simulink model "model2_2016a"  (R2016a)
settings: Solver=ode4  StartTime=0.0  StopTime=60  FixedStep=0.01  RelTol=1e-3
values from neighbouring files (symbols this model uses):
  D1 = par(2)    [cel.m]    (also in cel_P.m; cel_PD2.m = 38.2416; dane.m; dane.mat = 35.0184631454)
  D2 = par(4)    [cel.m]    (also in cel_P.m; cel_PD2.m = par(2); cel_z.m = par(2); dane.m)
  I3 = par(6)    [cel.m]    (also in cel_PD2.m = 0.0358; cel_bezFeedforward.m = par(2); dane.m; dane.mat = 0.0341130667622)
  Ko = 2    [dane.m]    (also in dane.mat = 10; dane2.mat = 10; dane3.mat = 10; dane4.mat = 10)
  Kr = par(7)    [cel.m]    (also in cel_P.m = par(5); cel_PD2.m = 0.3949; cel_bezFeedforward.m = par(3); dane.m = 3)
  Kw1 = 2    [dane.m]    (also in dane.mat = 10; dane2.mat = 10; dane3.mat = 10; dane4.mat = 10)
  Kw2 = 3    [dane.m]    (also in dane.mat = 5; dane2.mat = 5; dane3.mat = 5; dane4.mat = 5)
  limit2 = 10    [dane.m]    (also in dane.mat = 40; dane2.mat = 40; dane3.mat = 40; dane4.mat = 40)
  P1 = par(1)    [cel.m]    (also in cel_P.m; cel_PD2.m = 0.0302; dane.m; dane.mat = 0.804768322622)
  P2 = par(3)    [cel.m]    (also in cel_P.m; cel_PD2.m = par(1); cel_z.m = par(1); dane.m)
  P3 = par(5)    [cel.m]    (also in cel_PD2.m = 6.71669750093e-06; cel_bezFeedforward.m = par(1); dane.m; dane.mat = 3.3559799843e-06)
  r = 3    [dane.m]    (also in dane.mat = 50; dane2.mat = 20; dane3.mat = 70; dane4.mat = 70)
  tau = 0    [dane.m]    (also in dane.mat = 1; dane2.mat = 1; dane3.mat = 1; dane4.mat = 1)
  To = 2    [dane.m]    (also in dane.mat = 1; dane2.mat = 1; dane3.mat = 1; dane4.mat = 1)
  Tw2 = .1    (= 0.1)    [dane.m]    (also in dane.mat; dane2.mat; dane3.mat; dane4.mat)
undefined symbols (not defined in the file or in its folder): sigbuilder_block
libraries: simulink x2
settings Model: Creator=Maciek  LastModifiedBy=Daniel Rubak
settings GRTTargetCC: GeneratePreprocessorConditionals=Use local settings

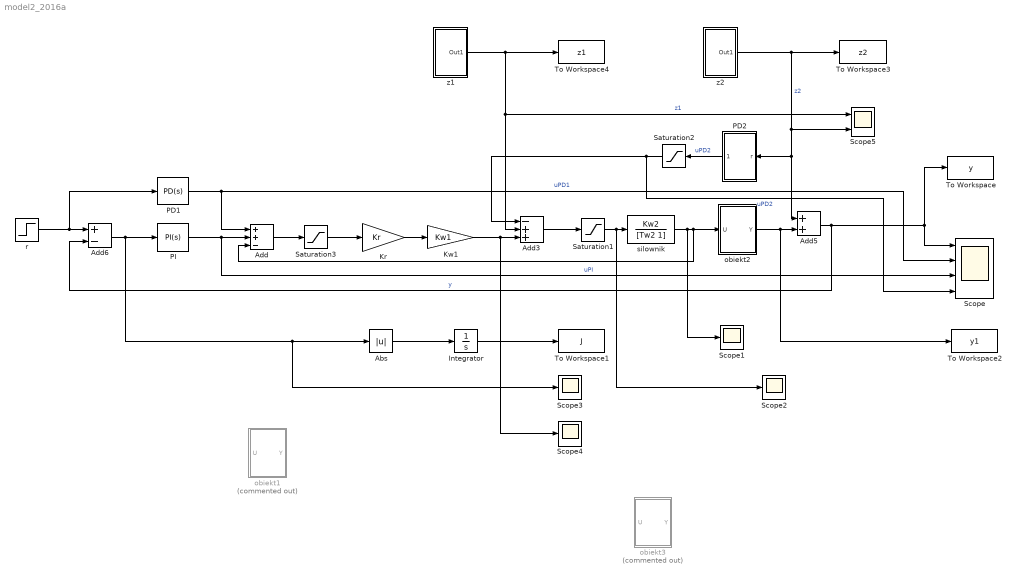
== system model2_2016a ==
  Abs : Abs
  Add : Sum  Inputs=++-
  Add3 : Sum  Inputs=-++
  Add5 : Sum
  Add6 : Sum  Inputs=+-
  Integrator : Integrator
  Kr : Gain  Gain=Kr
  "Kw1 " : Gain  Gain=Kw1
  PD1 : simulink/Continuous/PID Controller  Controller=PD  TimeDomain=Continuous-time  SampleTime=-1  IntegratorMethod=Forward Euler  FilterMethod=Forward Euler  Form=Parallel  UseFilter=on  ControllerParametersSource=internal  P=P1  I=1  D=D1  N=100  InitialConditionSource=internal  InitialConditionForIntegrator=0  InitialConditionForFilter=0  ExternalReset=none  LimitOutput=on  UpperSaturationLimit=limit2  LowerSaturationLimit=-limit2  LinearizeAsGain=on  AntiWindupMode=none  Kb=1  TrackingMode=off  Kt=1  PParamMin=[]  PParamMax=[]  IParamMin=[]  IParamMax=[]  DParamMin=[]  DParamMax=[]  NParamMin=[]  NParamMax=[]  KbParamMin=[]  KbParamMax=[]  KtParamMin=[]  KtParamMax=[]  POutMin=[]  POutMax=[]  IOutMin=[]  IOutMax=[]  DOutMin=[]  DOutMax=[]  NOutMin=[]  NOutMax=[]  KbOutMin=[]  KbOutMax=[]  KtOutMin=[]  KtOutMax=[]  IntegratorOutMin=[]  IntegratorOutMax=[]  FilterOutMin=[]  FilterOutMax=[]  SumOutMin=[]  SumOutMax=[]  SumI1OutMin=[]  SumI1OutMax=[]  SumI2OutMin=[]  SumI2OutMax=[]  SumI3OutMin=[]  SumI3OutMax=[]  SumDOutMin=[]  SumDOutMax=[]  SaturationOutMin=[]  SaturationOutMax=[]  IntegratorContinuousStateAttributes=''  IntegratorStateMustResolveToSignalObject=off  IntegratorRTWStateStorageClass=Auto  FilterContinuousStateAttributes=''  FilterStateMustResolveToSignalObject=off  FilterRTWStateStorageClass=Auto  DifferentiatorICPrevScaledInput=0  DifferentiatorOutMin=[]  DifferentiatorOutMax=[]
  PD2 : Subsystem
  PI : simulink/Continuous/PID Controller  Controller=PI  TimeDomain=Continuous-time  SampleTime=-1  IntegratorMethod=Forward Euler  FilterMethod=Forward Euler  Form=Parallel  UseFilter=on  ControllerParametersSource=internal  P=P3  I=I3  D=0  N=100  InitialConditionSource=internal  InitialConditionForIntegrator=0  InitialConditionForFilter=0  ExternalReset=none  LimitOutput=on  UpperSaturationLimit=limit2  LowerSaturationLimit=-limit2  LinearizeAsGain=on  AntiWindupMode=back-calculation  Kb=1/sqrt(max(0.001,I3))  TrackingMode=off  Kt=1  PParamMin=[]  PParamMax=[]  IParamMin=[]  IParamMax=[]  DParamMin=[]  DParamMax=[]  NParamMin=[]  NParamMax=[]  KbParamMin=[]  KbParamMax=[]  KtParamMin=[]  KtParamMax=[]  POutMin=[]  POutMax=[]  IOutMin=[]  IOutMax=[]  DOutMin=[]  DOutMax=[]  NOutMin=[]  NOutMax=[]  KbOutMin=[]  KbOutMax=[]  KtOutMin=[]  KtOutMax=[]  IntegratorOutMin=[]  IntegratorOutMax=[]  FilterOutMin=[]  FilterOutMax=[]  SumOutMin=[]  SumOutMax=[]  SumI1OutMin=[]  SumI1OutMax=[]  SumI2OutMin=[]  SumI2OutMax=[]  SumI3OutMin=[]  SumI3OutMax=[]  SumDOutMin=[]  SumDOutMax=[]  SaturationOutMin=[]  SaturationOutMax=[]  IntegratorContinuousStateAttributes=''  IntegratorStateMustResolveToSignalObject=off  IntegratorRTWStateStorageClass=Auto  FilterContinuousStateAttributes=''  FilterStateMustResolveToSignalObject=off  FilterRTWStateStorageClass=Auto  DifferentiatorICPrevScaledInput=0  DifferentiatorOutMin=[]  DifferentiatorOutMax=[]
  Saturation1 : Saturate  UpperLimit=limit2  LowerLimit=-limit2
  Saturation2 : Saturate  UpperLimit=20  LowerLimit=-20
  Saturation3 : Saturate  UpperLimit=limit2  LowerLimit=-limit2
  Scope : Scope  NumInputPorts=4
  Scope{1..4} (4 alike) : Scope
  Scope5 : Scope  NumInputPorts=2
  To Workspace : ToWorkspace  VariableName=y  SaveFormat=Timeseries  SampleTime=-1
  To Workspace1 : ToWorkspace  VariableName=J  SampleTime=-1
      settings: MaxDataPoints=1
  To Workspace2 : ToWorkspace  VariableName=y1  SaveFormat=Timeseries  SampleTime=-1
  To Workspace3 : ToWorkspace  VariableName=z2  SaveFormat=Timeseries  SampleTime=-1
  To Workspace4 : ToWorkspace  VariableName=z1  SaveFormat=Timeseries  SampleTime=-1
  obiekt1 : Subsystem  Commented=on
  obiekt2 : Subsystem
  obiekt3 : Subsystem  Commented=on
  r : Step  After=r  SampleTime=0
  silownik : TransferFcn  Numerator=Kw2  Denominator=[Tw2 1]
  z1 : Subsystem
  z2 : Subsystem
  wires:
  r/1 -> PD1/1, Add6/1
  PD1/1 -> Scope/2, Add/1  "uPD1"
  Kr/1 -> "Kw1 "/1
  PI/1 -> Add/2, Scope/3  "uPI"
  Add6/1 -> Scope3/1, Abs/1, PI/1
  Add5/1 -> Add6/2, To Workspace/1, Scope/1  "y"
  PD2/1(uPD2) -> Saturation2/1  "uPD2"
  obiekt2/1(Y) -> To Workspace2/1, Add5/2
  Integrator/1 -> To Workspace1/1
  Abs/1 -> Integrator/1
  Saturation1/1 -> Scope2/1, silownik/1
  Saturation2/1 -> Scope/4, Add3/1  "uPD2"
  Add3/1 -> Saturation1/1
  z1/1(Out1) -> Scope5/1, Add3/2, To Workspace4/1  "z1"
  z2/1(Out1) -> To Workspace3/1, Scope5/2, Add5/1, PD2/1(r)  "z2"
  "Kw1 "/1 -> Scope4/1, Add3/3
  Saturation3/1 -> Kr/1
  silownik/1 -> Scope1/1, obiekt2/1(U), Add/3
  Add/1 -> Saturation3/1

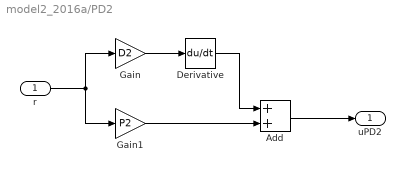
== system model2_2016a/PD2 ==
  r : Inport
  Add : Sum
  Derivative : Derivative
  Gain : Gain  Gain=D2
  Gain1 : Gain  Gain=P2
  uPD2 : Outport
  wires:
  Derivative/1 -> Add/1
  Gain1/1 -> Add/2
  r/1 -> Gain/1, Gain1/1
  Gain/1 -> Derivative/1
  Add/1 -> uPD2/1

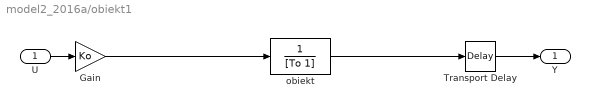
== system model2_2016a/obiekt1 ==
  U : Inport
  Gain : Gain  Gain=Ko
  Transport Delay : TransportDelay  DelayTime=tau
  obiekt : TransferFcn  Numerator=1  Denominator=[To 1]
  Y : Outport
  wires:
  U/1 -> Gain/1
  Gain/1 -> obiekt/1
  Transport Delay/1 -> Y/1
  obiekt/1 -> Transport Delay/1

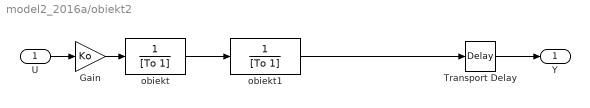
== system model2_2016a/obiekt2 ==
  U : Inport
  Gain : Gain  Gain=Ko
  Transport Delay : TransportDelay  DelayTime=tau
  obiekt : TransferFcn  Numerator=1  Denominator=[To 1]
  obiekt1 : TransferFcn  Numerator=1  Denominator=[To 1]
  Y : Outport
  wires:
  U/1 -> Gain/1
  Gain/1 -> obiekt/1
  obiekt/1 -> obiekt1/1
  Transport Delay/1 -> Y/1
  obiekt1/1 -> Transport Delay/1

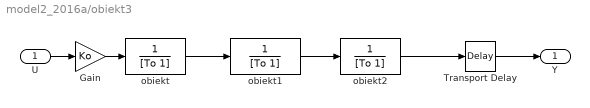
== system model2_2016a/obiekt3 ==
  U : Inport
  Gain : Gain  Gain=Ko
  Transport Delay : TransportDelay  DelayTime=tau
  obiekt : TransferFcn  Numerator=1  Denominator=[To 1]
  obiekt1 : TransferFcn  Numerator=1  Denominator=[To 1]
  obiekt2 : TransferFcn  Numerator=1  Denominator=[To 1]
  Y : Outport
  wires:
  U/1 -> Gain/1
  Gain/1 -> obiekt/1
  obiekt/1 -> obiekt1/1
  obiekt1/1 -> obiekt2/1
  Transport Delay/1 -> Y/1
  obiekt2/1 -> Transport Delay/1

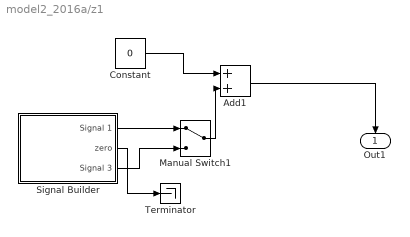
== system model2_2016a/z1 ==
  Add1 : Sum
  Constant : Constant  Value=0
  Manual Switch1 : ManualSwitch
  Signal Builder : Subsystem  Tag=STV Subsys  LoadFcn=sigbuilder_block('load');  StartFcn=sigbuilder_block('start');  StopFcn=sigbuilder_block('stop');  ClipboardFcn=sigbuilder_block('clipboard');  mask(Sigbuilder block){}
      mask help: Simulink:masks:SigbuilderBlock_MD
      mask init:
      | if ~strcmp(get_param(bdroot(gcbh),'SimulationStatus'),'stopped') tuvar = sigbuilder_block('maskInit'); end
      settings: CopyFcn=sigbuilder_block('copy');  DeleteFcn=sigbuilder_block('delete');  ModelCloseFcn=sigbuilder_block('modelClose');  PreSaveFcn=sigbuilder_block('preSave');  PauseFcn=sigbuilder_block('pause');  ContinueFcn=sigbuilder_block('continue');  NameChangeFcn=sigbuilder_block('namechange');  OpenFcn=sigbuilder_block('open',[1542.6 -54.6 1012.8 448.2 ]);  CloseFcn=sigbuilder_block('close');
      mask Display: plot(0, 0, 100, 100,[2, 2, 32, 32, 2], [68, 8, 8, 68, 68],[32, 2], [38, 38], [32, 19, 2],[53, 60, 44], [32, 17, 17, 2],[16, 16, 31, 31]);txt = getActiveGroup(gcbh);text(2, 100, txt,'verticalAlignment', 'top');
  Terminator : Terminator
  Out1 : Outport
  wires:
  Signal Builder/1(Signal 1) -> Manual Switch1/1
  Signal Builder/3(Signal 3) -> Manual Switch1/2
  Signal Builder/2(zero) -> Terminator/1
  Manual Switch1/1 -> Add1/2
  Constant/1 -> Add1/1
  Add1/1 -> Out1/1

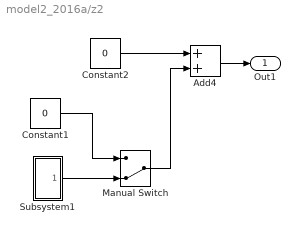
== system model2_2016a/z2 ==
  Add4 : Sum
  Constant1 : Constant  Value=0
  Constant2 : Constant  Value=0
  Manual Switch : ManualSwitch  CurrentSetting=0
  Subsystem1 : Subsystem
  Out1 : Outport
  wires:
  Subsystem1/1(Out1) -> Manual Switch/2
  Constant1/1 -> Manual Switch/1
  Add4/1 -> Out1/1
  Constant2/1 -> Add4/1
  Manual Switch/1 -> Add4/2

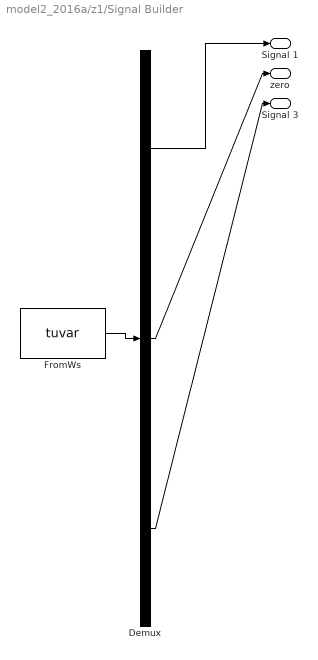
== system model2_2016a/z1/Signal Builder ==
  Demux : Demux  Tag=STV Demux  Outputs=3
  FromWs : FromWorkspace  Tag=STV FromWs  VariableName=tuvar  SampleTime=0.01
      SigBuilderData=|
      | common.afterFinalStr = 'Extrapolate'
      | common.sampleTime = '0.01'
      | dataSet.timeRange = [0 60]
      | dataSet.name = 'Group 1'
      | sbobj.Groups.Name = 'Group 1'
      | sbobj.Groups.Signals(1).Name = 'Signal 1'
      | sbobj.Groups.Signals(1).XData = [0 10 15 15 17 17 40 40 43 43 60]
      | sbobj.Groups.Signals(1).YData = [0 0 0 1 1 0 0 -1.5 -1.5 0 0]
      | sbobj.Groups.Signals(2).Name = 'zero'
      | sbobj.Groups.Signals(2).XData = [0 15 17 25 29 40 60]
      | sbobj.Groups.Signals(2).YData = [0 0 0 0 0 0 0]
      | sbobj.Groups.Signals(3).Name = 'Signal 3'
      | sbobj.Groups.Signals(3).XData = [0 4 5 9 15 15 17 17 25 25 29 29 35 36 40 40 43 43 49 50 54 55 60]
      | sbobj.Groups.Signals(3).YData = [0 0 0 0 0 1 1 0 0 -4 -4 0 0 0 0 1 1 0 0 0 0 0 0]
      | sbobj.Groups.TimeRange = [0 60]
  Signal 1 : Outport  Tag=STV Outport
  zero : Outport  Tag=STV Outport  Port=2
  Signal 3 : Outport  Tag=STV Outport  Port=3
  wires:
  Demux/1 -> Signal 1/1
  FromWs/1 -> Demux/1
  Demux/2 -> zero/1
  Demux/3 -> Signal 3/1

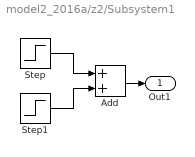
== system model2_2016a/z2/Subsystem1 ==
  Add : Sum
  Step : Step  Time=20  After=5  SampleTime=0
  Step1 : Step  Time=30  After=-5  SampleTime=0
  Out1 : Outport
  wires:
  Add/1 -> Out1/1
  Step/1 -> Add/1
  Step1/1 -> Add/2
